simulink model "CubeSat_ADCS"  (R2026a)
settings: Solver=ode4  StopTime=tfinal  FixedStep=1
values from neighbouring files (symbols this model uses):
  A = 0.02    [magnetorquer_params.m]
  Amax = lsort(2)*lsort(3)    [inertia.m]
  AngBias = [1e-4; -2e-4; 1e-4]    [sensor_params.m]
  AngNoise = 1e-4    (= 0.0001)    [sensor_params.m]
  CD = 1.0    (= 1)    [inertia.m]
  desatSpeed = rpm_desat*2*pi/60    (= 104.71975512)    [reaction_wheel_params.m]
  G = 6.67e-11    [planet_params.m]
  Ir1B = T1*IrR*T1'    [reaction_wheel_params.m]
  Ir1Bcg = Ir1B + m_rws*(sr1')*sr1    [reaction_wheel_params.m]
  Ir2B = T2*IrR*T2'    [reaction_wheel_params.m]
  Ir2Bcg = Ir2B + m_rws*(sr2')*sr2    [reaction_wheel_params.m]
  Ir3B = T3*IrR*T3'    [reaction_wheel_params.m]
  Ir3Bcg = Ir3B + m_rws*(sr3')*sr3    [reaction_wheel_params.m]
  Is = (ms/12)*[(ly^2+lz^2) 0 0 ;0 (lx^2+lz^2) 0;0 0 (lx^2+ly^2)]    [inertia.m]
  Jinv = J'/(J*J')    [reaction_wheel_params.m]
  k = 0.001    [Control.m]    (also in Init_Params.m = 67200; main_final.m = (1/6)*(k1+2*k2+2*k3+k4))
  lmax = l(3)    [inertia.m]
  m = ms + 3*m_rws    [inertia.m]
  M = 5.972e24    (= 5.972e+24)    [planet_params.m]
  MagBias = [1e-7; -2e-7; 1.5e-7]    [sensor_params.m]
  MagNoise = 1e-6    (= 1e-06)    [sensor_params.m]
  maxAlpha = maxTorque/IrR(1,1)    [reaction_wheel_params.m]
  maxSpeed = max_rpm*2*pi/60    (= 733.038285838)    [reaction_wheel_params.m]
  n = 84    [magnetorquer_params.m]
  n1 = [1;0;0]    [reaction_wheel_params.m]
  n2 = [0;1;0]    [reaction_wheel_params.m]
  n3 = [0;0;1]    [reaction_wheel_params.m]
  pqr0 = [0.08; -0.02; 0.03]    [Init_Params.m]    (also in main_final.m = [p0; q0; r0])
  q0 = q0123(1)    [Body2ECI_quat.m]    (also in EulerAngles2Quaternions.m = cos(phi/2)*cos(theta/2)*cos(psi/2) + sin(phi/2)*sin(theta/2); Init_Params.m = EulerAngles2Quaternions(ptp0); Quaternions2EulerAngles.m = q0123(:,1); main_final.m = -0.02)
  r0_eci = [x0; y0; z0]    [Init_Params.m]
  s = 0.3    [Init_Params.m]    (also in Navigation.m)
  v0_eci = [0; vcircular*cos(inclination); vcircular*sin(inclination)]    [Init_Params.m]
undefined symbols (not defined in the file or in its folder): IAU
libraries: matrix_library x4, aerolibtransform2 x3, vrlib x3, simulink x3, aerolibutil x1, simulink_extras x1
settings Model: Creator=marca  LastModifiedBy=marca
settings DebuggingCC: SignalInfNanChecking=warning  UnderSpecifiedDimensionMsg=warning

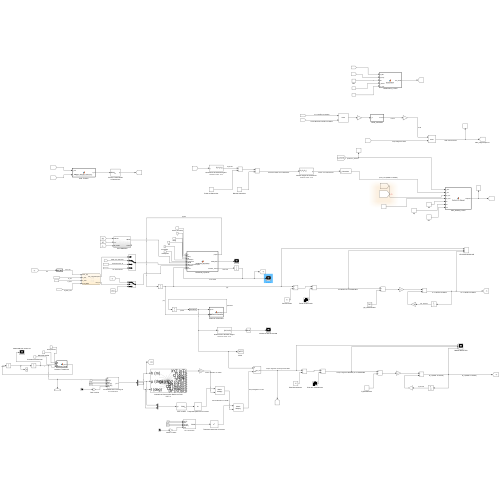
[thumbnail: Simulink's stored preview of the top-level diagram]
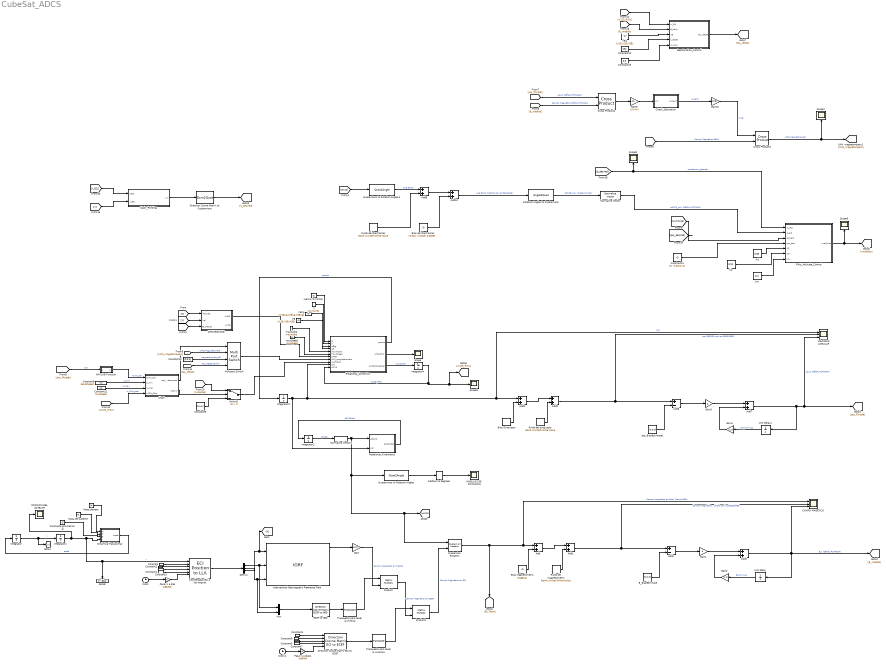
== system CubeSat_ADCS ==
  Add{,1..3,5,7,9..10} (8 alike) : Sum
  Add4 : Sum  Inputs=+-
  Add6 : Sum  Inputs=+-
  B_BiasEstimate : Constant  Value=[0;0;0]
  Bias Giroscopio : Constant  Value=AngBias
  Bias Magnetómetro : Constant  Value=MagBias
  Bias del Startracker : Constant  Value=[0.001; -0.0015; 0.0008]
  CAMPO MAGÉTICO : Scope  NumInputPorts=3
      settings: ActiveDisplayYMinimum=-5.4427960375962918E-5  ActiveDisplayYMaximum=3.9521146554244587E-5  DataLoggingVariableName=ScopeData4
  Chart : Stateflow chart  TreatAsAtomicUnit=on
  Check_Saturation : MATLAB Function  TreatAsAtomicUnit=on
  Clock : Clock
  Clock1 : Clock
  Constant : Constant  Value=0  SampleTime=-1
  Constant{1,3,5,7} (4 alike) : Constant  Value=[0,0]
  Constant10 : Constant  Value=[0;0;0]
  Constant11 : Constant  Value=maxSpeed
  Constant12 : Constant  Value=1e4
  Constant13 : Constant  Value=0.5
  Constant14 : Constant  Value=[0; -0.0011; 0]
  Constant2 : Constant  Value=0
  Constant4 : Constant  Value=0
  Constant6 : Constant  Value=0
  Constant8 : Constant  Value=desatSpeed
  Constant9 : Constant  Value=[0;0;0]
  Constante gravitacional : Constant  Value=G
  Coordenadas ECI a lat-long-alt : aerolibtransform2/ECI Position to LLA  red=IAU-2000/2006  year=2026  month=August  day=1  hour=0  min=0  sec=0  deltaT=Day  errorflag=Error  extraparamflag=on  eunits=Metric (MKS)  earthmodel=WGS84  flat=1/298.257223563  eqradius=6378137
      settings: AttributesFormatString=%<red>
  Cross Product2 : matrix_library/Cross Product
  Cross Product3 : matrix_library/Cross Product
  DISTURBANCE : Subsystem
  Demux : Demux  Outputs=3
  Desaturation_Control : MATLAB Function  TreatAsAtomicUnit=on
  Dinámica Traslacional : MATLAB Function  TreatAsAtomicUnit=on
  Direction Cosine Matrix ECI to ECEF : aerolibtransform2/Direction Cosine Matrix ECI to ECEF  red=IAU-2000/2006  year=2026  month=August  day=1  hour=0  min=0  sec=0  deltaT=Day  errorflag=Error  extraparamflag=on
      settings: AttributesFormatString=%<red>
  Direction Cosine Matrix to Quaternions : Dcm2Quat
  ECEF to NED : aerolibtransform2/Direction Cosine Matrix ECEF to NED
  Gain : Gain  Gain=1e-9
  Gain1 : Gain  Gain=s
  Gain10 : Gain  Gain=n*A
  Gain2 : Gain  Gain=(1-s)
  Gain3 : Gain  Gain=s
  Gain4 : Gain  Gain=(1-s)
  Gain9 : Gain  Gain=k/(n*A)
  Inercia (sin RWs) : Constant  Value=Is
  Integrator : Integrator  InitialCondition=v0_eci
  Integrator1 : Integrator  InitialCondition=r0_eci
  Integrator2 : Integrator  InitialCondition=q0
  Integrator3 : Integrator  InitialCondition=pqr0
  Integrator4 : Integrator  InitialCondition=[0;0;0]
  International Geomagnetic Reference Field : IGRF  time_in=off  month=August  day=1  year=2026
      settings: AttributesFormatString=%<generation>
  IrB : Constant  Value=[Ir1B,Ir2B,Ir3B]
  IrB1 : Constant  Value=[Ir1B,Ir2B,Ir3B]
  IrBcg : Constant  Value=[Ir1Bcg,Ir2Bcg,Ir3Bcg]
  Jinv : Constant  Value=Jinv
  Kd : Constant  Value=0.05
  Kp : Constant  Value=0.01
  MATLAB Function : MATLAB Function  TreatAsAtomicUnit=on
  Masa del satélite : Constant  Value=m
  Masa planeta : Constant  Value=M
  Multiport Switch : MultiPortSwitch  SaturateOnIntegerOverflow=off  InputSameDT=off
  Mux : Mux  Inputs=2
  Nadir_Pointing : MATLAB Function  TreatAsAtomicUnit=on
  Normalize Vector : vrlib/Utilities/Normalize Vector  maxzero=0
  Normalize Vector1 : vrlib/Utilities/Normalize Vector  maxzero=0
  POSICIÓN DEL SATÉLITE : Scope
      settings: ActiveDisplayYMinimum=-8.7137499994663056E+6  ActiveDisplayYMaximum=8.7137499999407E+6
  Pasar s a dias : Gain  Gain=1/86400
  Pasar s a dias1 : Gain  Gain=1/86400
  Product : Product  Multiplication=Matrix(*)
  Product1 : Product  Multiplication=Matrix(*)
  Quaternion Rotation : aerolibutil/Quaternion Rotation
  Quaternions to Rotation Angles : Quat2Angle
      settings: AttributesFormatString=Rotation Order: %<rotationOrder>
  Quaternions to Rotation Angles1 : Quat2Angle
      settings: AttributesFormatString=Rotation Order: %<rotationOrder>
  RWs_Attitude_Control : MATLAB Function  TreatAsAtomicUnit=on
  Radians to Degrees : simulink_extras/Transformations/Radians to Degrees
  Rotation Angles to Quaternions : Angle2Quat
      settings: AttributesFormatString=Rotation Order: %<rotationOrder>
  Rotational_Dynamics : MATLAB Function  TreatAsAtomicUnit=on
  Rotational_Kinematics : MATLAB Function  TreatAsAtomicUnit=on
  Ruido del Startracker : simulink/Sources/Band-Limited White Noise  Cov=[9.4e-9; 9.4e-9; 2.3e-7]  Ts=1  seed=[23341]
  Ruido del giroscopio : simulink/Sources/Band-Limited White Noise  Cov=((AngNoise)^2) * [1; 1; 1]  Ts=1  seed=[23341]
  Ruido del magnetómetro : simulink/Sources/Band-Limited White Noise  Cov=(MagNoise^2) * [1; 1; 1]  Ts=1  seed=[23341]
  Scope{,1..3,5} (5 alike) : Scope
      Scope settings: ActiveDisplayYMinimum=-0.0029922508301770847  ActiveDisplayYMaximum=0.0037761427901097859
      Scope1 settings: ActiveDisplayYMinimum=-1.896452021703556E-8  ActiveDisplayYMaximum=1.737154328387897E-6  DataLoggingVariableName=ScopeData5
      Scope2 settings: ActiveDisplayYMinimum=-0.49886917310286244  ActiveDisplayYMaximum=-0.0070450072202054848  DataLoggingVariableName=ScopeData6
      Scope3 settings: ActiveDisplayYMinimum=-138.56846791071905  ActiveDisplayYMaximum=115.27734503606811  DataLoggingVariableName=ScopeData7
      Scope5 settings: ActiveDisplayYMinimum=-24.785061505875653  ActiveDisplayYMaximum=36.707156844753371  DataLoggingVariableName=ScopeData9
  Switch1 : Switch  Criteria=u2 > Threshold  SaturateOnIntegerOverflow=off  InputSameDT=off
  Traspuesta para tener la inversa : matrix_library/Transpose
  Traspuesta para tener la inversa1 : matrix_library/Transpose
  Unit Delay : UnitDelay  InitialCondition=[0;0;0]  SampleTime=-1
  Unit Delay1 : UnitDelay  InitialCondition=[0;0;0]  SampleTime=-1
  VELCIDAD ANGULAR : Scope  NumInputPorts=3
      settings: ActiveDisplayYMinimum=-0.3287242244754594  ActiveDisplayYMaximum=0.46714614565610874  DataLoggingVariableName=ScopeData3
  maxAlpha : Constant  Value=maxAlpha
  maxSpeed : Constant  Value=maxSpeed
  n : Constant  Value=[n1,n2,n3]
  pqr_BiasEstimate1 : Constant  Value=[0;0;0]
  ÁNGULOS DE ROTACIÓN : Scope
      settings: ActiveDisplayYMinimum=-82.561568673125265  ActiveDisplayYMaximum=52.799854649442857  DataLoggingVariableName=ScopeData2
  wires:
  Integrator/1 -> [v], Integrator1/1  "v"
  Dinámica Traslacional/1(accel) -> Integrator/1  "accel"
  Integrator1/1 -> POSICIÓN DEL SATÉLITE/1, Coordenadas ECI a lat-long-alt/1, [r_ECI], Dinámica Traslacional/4(r)  "r"
  Masa planeta/1 -> Dinámica Traslacional/1(M)
  Masa del satélite/1 -> Dinámica Traslacional/2(m)
  Constante gravitacional/1 -> Dinámica Traslacional/3(G)
  Integrator2/1 -> Normalize Vector1/1  "q0123"
  Inercia (sin RWs)/1 -> Rotational_Dynamics/1(Is)
  Rotational_Dynamics/1(pqrdot) -> Integrator3/1  "pqrdot"
  Integrator3/1 -> Rotational_Kinematics/2(pqr), VELCIDAD ANGULAR/1, Add2/1, Rotational_Dynamics/10(pqr)  "pqr"
  Rotational_Kinematics/1(q0123dot) -> Integrator2/1  "q0123dot"
  Quaternions to Rotation Angles/1 -> Radians to Degrees/1
  Coordenadas ECI a lat-long-alt/1 -> Demux/1
  Demux/1 -> Mux/1, International Geomagnetic Reference Field/2
  Demux/2 -> Mux/2, International Geomagnetic Reference Field/3
  Demux/3 -> [h], International Geomagnetic Reference Field/1
  Constant/1 -> Coordenadas ECI a lat-long-alt/2
  Constant2/1 -> Coordenadas ECI a lat-long-alt/3
  Constant3/1 -> Coordenadas ECI a lat-long-alt/4
  Constant1/1 -> Coordenadas ECI a lat-long-alt/5
  Clock/1 -> Pasar s a dias/1
  Pasar s a dias/1 -> Coordenadas ECI a lat-long-alt/6
  International Geomagnetic Reference Field/1 -> Gain/1
  Gain/1 -> Product/2  "Campo magnético en Teslas"
  Mux/1 -> ECEF to NED/1
  ECEF to NED/1 -> Traspuesta para tener la inversa/1
  Traspuesta para tener la inversa/1 -> Product/1
  Pasar s a dias1/1 -> Direction Cosine Matrix ECI to ECEF/5
  Constant7/1 -> Direction Cosine Matrix ECI to ECEF/3
  Constant4/1 -> Direction Cosine Matrix ECI to ECEF/1
  Constant6/1 -> Direction Cosine Matrix ECI to ECEF/2
  Constant5/1 -> Direction Cosine Matrix ECI to ECEF/4
  Clock1/1 -> Pasar s a dias1/1
  Direction Cosine Matrix ECI to ECEF/1 -> Traspuesta para tener la inversa1/1
  Product/1 -> Product1/2  "Campo Magnético en ECEF"
  Traspuesta para tener la inversa1/1 -> Product1/1
  Product1/1 -> Quaternion Rotation/2  "Campo Magnético en ECI"
  Quaternion Rotation/1 -> CAMPO MAGÉTICO/1, Add/1, [BI_Tesla]  "Campo magnético en Body Frame REAL"
  Bias Magnetómetro/1 -> Add/2
  Add/1 -> Add1/1
  Ruido del magnetómetro/1 -> Add1/2
  Add1/1 -> Add4/1, CAMPO MAGÉTICO/2  "Campo magnético MEDIDO por los SENSORES"
  Add2/1 -> Add3/1
  Ruido del giroscopio/1 -> Add3/2
  Add3/1 -> Add6/1, VELCIDAD ANGULAR/2  "pqr MEDIDA por los SENSORES"
  Bias Giroscopio/1 -> Add2/2
  B_BiasEstimate/1 -> Add4/2
  Add4/1 -> Gain1/1
  Unit Delay/1 -> Gain2/1  "B_kminus1"
  Gain2/1 -> Add5/2
  Gain1/1 -> Add5/1
  Add5/1 -> [B_medido], CAMPO MAGÉTICO/3, Unit Delay/1  "B_k (SEÑAL FILTRADA)"
  Gain4/1 -> Add7/2
  Unit Delay1/1 -> Gain4/1  "pqr_kminus1"
  Add7/1 -> VELCIDAD ANGULAR/3, [pqr_filtrada], Unit Delay1/1  "pqr_k (SEÑAL FILTRADA)"
  pqr_BiasEstimate1/1 -> Add6/2
  Add6/1 -> Gain3/1
  Gain3/1 -> Add7/1
  maxAlpha/1 -> Rotational_Dynamics/5(maxAlpha)
  n/1 -> Rotational_Dynamics/2(n)
  IrB/1 -> Rotational_Dynamics/4(IrB)
  IrBcg/1 -> Rotational_Dynamics/3(IrBcg)
  Rotational_Dynamics/3(w123dot_actual) -> Integrator4/1  "w123_dot"
  Integrator4/1 -> [w123_RWs], Scope3/1, Rotational_Dynamics/11(w123)  "w123_RWs"
  [h] -> DISTURBANCE/1(Altitude)
  [v] -> DISTURBANCE/2(vel)
  [BI_Tesla] -> DISTURBANCE/3(BI_Teslas)
  [q0123] -> Quaternions to Rotation Angles1/1
  Ruido del Startracker/1 -> Add9/2
  Quaternions to Rotation Angles1/1 -> Add9/1  "Ang Euler"
  Add9/1 -> Add10/1
  Bias del Startracker/1 -> Add10/2
  Add10/1 -> Rotation Angles to Quaternions/1  "Ang Euler medido por el Startracker"
  Rotation Angles to Quaternions/1 -> Normalize Vector/1  "q0123_nav (cuaterniones)"
  Normalize Vector/1 -> RWs_Attitude_Control/2(q_act)  "q0123_nav (SEÑAL FILTRADA)"
  [pqr_filtrada] -> RWs_Attitude_Control/3(pqr_act)
  Gain10/1 -> Cross Product3/1  "muB"
  Cross Product3/1 -> Scope1/1, [LMN_magnetorquers]  "LMN_magnetorquers"
  Check_Saturation/1(current) -> Gain10/1  "current"
  [pqr_filtrada] -> Cross Product2/1  "pqr_k (SEÑAL FILTRADA)"
  Gain9/1 -> Check_Saturation/1(i_in)
  Cross Product2/1 -> Gain9/1
  [B_medido] -> Cross Product2/2  "Campo Magnético SEÑAL FILTRADA"
  [BI_Tesla] -> Cross Product3/2  "Campo Magnético REAL"
  Rotational_Dynamics/2(LMN_RWs) -> Scope/1
  maxSpeed/1 -> Rotational_Dynamics/6(maxSpeed)
  DISTURBANCE/1(LMND) -> Rotational_Dynamics/7(LMND)
  [q_desired] -> RWs_Attitude_Control/1(q_des), Scope2/1  "quaternion_desired"
  Radians to Degrees/1 -> ÁNGULOS DE ROTACIÓN/1
  [pqr_filtrada] -> MATLAB Function/1(pqr_filtrada)  "pqr"
  MATLAB Function/1(norm_pqr) -> Chart/1(norm_pqr)  "norm_pqr"
  Chart/2(use_rw) -> Switch1/2
  [LMN_magnetorquers] -> Multiport Switch/2  "LMN_mag_detumble"
  [rwalphas] -> Switch1/1
  Constant9/1 -> Switch1/3
  Multiport Switch/1 -> Rotational_Dynamics/8(LMN_magnetorquers)
  Switch1/1 -> Rotational_Dynamics/9(rwalphas)
  [w123_RWs] -> Chart/4(w123_RWs)  "w_RWs_real"
  Constant8/1 -> Chart/2(w_min)  "w_min"
  Constant11/1 -> Chart/3(w_max)  "w_max"
  Chart/1(use_magnetorquers) -> Multiport Switch/1
  Constant10/1 -> Multiport Switch/3  "magnetorquers_off"
  [w123_RWs] -> Desaturation_Control/1(w_RW)
  [B_medido] -> Desaturation_Control/2(B_body)
  IrB1/1 -> Desaturation_Control/3(IrB)
  Constant12/1 -> Desaturation_Control/4(k_desat)
  Constant13/1 -> Desaturation_Control/5(m_max)
  Desaturation_Control/1(tau_desat) -> [tau_desat]
  [tau_desat] -> Multiport Switch/4  "tau_desaturación"
  [r_ECI] -> Nadir_Pointing/1(r_ECI)
  [v] -> Nadir_Pointing/2(v_ECI)
  [pqr_desired] -> ?
  Normalize Vector1/1 -> Rotational_Kinematics/1(q0123), [q0123], Quaternion Rotation/1, Quaternions to Rotation Angles/1
  Constant14/1 -> RWs_Attitude_Control/4(pqr_des)
  Nadir_Pointing/1(xyz) -> Direction Cosine Matrix to Quaternions/1
  Direction Cosine Matrix to Quaternions/1 -> [q_desired]
  Kd/1 -> RWs_Attitude_Control/5(KP)
  Jinv/1 -> RWs_Attitude_Control/7(Jinv)
  Kp/1 -> RWs_Attitude_Control/6(KD)
  RWs_Attitude_Control/1(rwalphas) -> Scope5/1, [rwalphas]

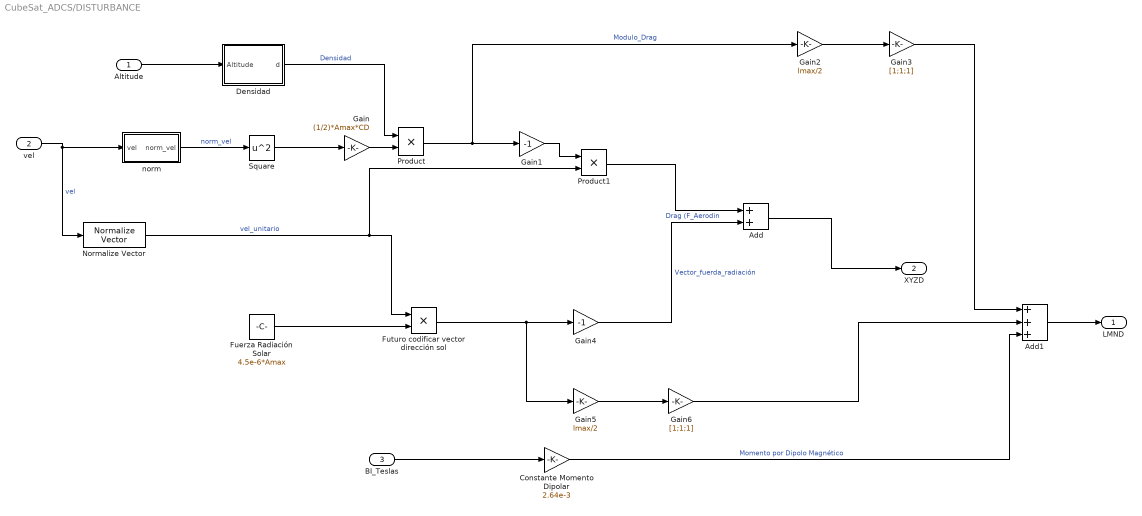
== system CubeSat_ADCS/DISTURBANCE ==
  Altitude : Inport
  vel : Inport  Port=2
  BI_Teslas : Inport  Port=3
  Add : Sum
  Add1 : Sum  Inputs=+++
  Constante Momento Dipolar : Gain  Gain=2.64e-3
  Densidad : MATLAB Function  TreatAsAtomicUnit=on
  Fuerza Radiación Solar : Constant  Value=4.5e-6*Amax
  Futuro codificar vector dirección sol : Product
  Gain : Gain  Gain=(1/2)*Amax*CD
  Gain1 : Gain  Gain=-1
  Gain2 : Gain  Gain=lmax/2
  Gain3 : Gain  Gain=[1;1;1]
  Gain4 : Gain  Gain=-1
  Gain5 : Gain  Gain=lmax/2
  Gain6 : Gain  Gain=[1;1;1]
  Normalize Vector : vrlib/Utilities/Normalize Vector  maxzero=0
  Product : Product
  Product1 : Product
  Square : Math  Operator=square
  norm : MATLAB Function  TreatAsAtomicUnit=on
  LMND : Outport
  XYZD : Outport  Port=2
  wires:
  Altitude/1 -> Densidad/1(Altitude)
  vel/1 -> norm/1(vel), Normalize Vector/1  "vel"
  Normalize Vector/1 -> Futuro codificar vector dirección sol/1, Product1/2  "vel_unitario"
  Gain/1 -> Product/2
  norm/1(norm_vel) -> Square/1  "norm_vel"
  Square/1 -> Gain/1
  Product/1 -> Gain2/1, Gain1/1  "Modulo_Drag"
  Product1/1 -> Add/1  "Drag (F_Aerodin"
  Gain1/1 -> Product1/1
  Add/1 -> XYZD/1
  Gain2/1 -> Gain3/1
  Gain3/1 -> Add1/1
  Add1/1 -> LMND/1
  Fuerza Radiación Solar/1 -> Futuro codificar vector dirección sol/2
  Futuro codificar vector dirección sol/1 -> Gain5/1, Gain4/1
  Gain4/1 -> Add/2  "Vector_fuerda_radiación"
  Gain5/1 -> Gain6/1
  Gain6/1 -> Add1/2
  BI_Teslas/1 -> Constante Momento Dipolar/1
  Constante Momento Dipolar/1 -> Add1/3  "Momento por Dipolo Magnético"
  Densidad/1(d) -> Product/1  "Densidad"

== matlab function CubeSat_ADCS/Nadir_Pointing ==
  data: r_ECI input; xyz output; v_ECI input
function xyz  = Nadir_Attitude_Reference(r_ECI,v_ECI)

%%% NADIR PONTING %%%
% Se tomará el eje +Z como Nadir, el eje Y perpendicular al plano orbital 
% y el eje Z perpendicular a los dos ejes anteriores. 

z = -r_ECI/norm(r_ECI);

y = cross(z, v_ECI);
y = y / norm(y);

x = cross(z,y);

xyz = [x'; y'; z'];

== matlab function CubeSat_ADCS/RWs_Attitude_Control ==
  data: q_des input; rwalphas output; q_act input; pqr_act input; pqr_des input; KP input; KD input; Jinv input
function rwalphas = Control_PD_Robust(q_des, q_act, pqr_act, pqr_des, KP, KD, Jinv)
% 1. Normalización
q_des = q_des / norm(q_des);
q_act = q_act / norm(q_act);

% Asumiendo formato Scalar-First [q0; q1; q2; q3]
q0_d = q_des(1); qv_d = q_des(2:4);
q0_a = q_act(1); qv_a = q_act(2:4);

% 2. Cuaternión Error (q_error = q_des^-1 * q_act)
q0_err = q0_d * q0_a + dot(qv_d, qv_a);
qv_err = q0_d * qv_a - q0_a * qv_d - cross(qv_d, qv_a);

% 3. Corrección Anti-Discontinuidad (Shortest Path)
if q0_err < 0
    qv_err = -qv_err;
end
   
% 4. Error de velocidad angular
pqr_err = pqr_act - pqr_des;

% 5. Par de control y aceleración de ruedas
tau_cmd = - KP * qv_err - KD * pqr_err;
rwalphas = - Jinv * tau_cmd;

== matlab function CubeSat_ADCS/Rotational_Kinematics ==
  data: q0123 input; q0123dot output; pqr input
function q0123dot = Rotational_kinematics(q0123, pqr)
p = pqr(1); q= pqr(2); r = pqr(3);
PQRMAT = [0 -p -q -r;p 0 r -q; q -r 0 p; r q -p 0];
q0123dot = (1/2)*PQRMAT*q0123;

== matlab function CubeSat_ADCS/Dinámica Traslacional ==
  data: M input; m input; G input; r input; accel output
function accel = Translational_Dynamics(M,m,G,r)
r = r(:);
rho = norm(r);
r_unit = r/rho; 
Fgrav = -(G*M*m/rho^2)*r_unit; 

accel = Fgrav/m;

== matlab function CubeSat_ADCS/Rotational_Dynamics ==
  data: pqrdot output size=[3 1]; LMN_RWs output size=[3 1]; w123dot_actual output size=[3 1]; Is input size=[3 3]; n input size=[3 3]; IrBcg input size=[3 9]; IrB input size=[3 9]; maxAlpha input size=[1 1]; maxSpeed input; LMND input size=[3 1]; LMN_magnetorquers input size=[3 1]; rwalphas input size=[3 1]; pqr input size=[3 1]; w123 input size=[3 1]
function [pqrdot, LMN_RWs, w123dot_actual] = Rotational_Dynamics(Is, n, IrBcg, IrB, maxAlpha,maxSpeed,LMND,LMN_magnetorquers,rwalphas,pqr,w123)

% Pre-asignación para asegurar dimensiones fijas 3x1 en Simulink
pqrdot = zeros(3,1);
LMN_RWs = zeros(3,1);
w123dot_actual = zeros(3,1);

% Vectores de dirección (3x1)
n1 = n(:,1);
n2 = n(:,2);
n3 = n(:,3);

% Extraer las MATRICES 3x3 completas desde las entradas 3x9
Ir1B = IrB(:, 1:3);
Ir2B = IrB(:, 4:6);
Ir3B = IrB(:, 7:9);

Ir1Bcg = IrBcg(:, 1:3);
Ir2Bcg = IrBcg(:, 4:6);
Ir3Bcg = IrBcg(:, 7:9);

% Inercia total sumada (3x3)
I = Is + Ir1Bcg + Ir2Bcg + Ir3Bcg;
invI = inv(I);

% Limitación de aceleración por hardware
% Limitación de aceleración y velocidad por hardware (CORREGIDO)
for idx = 1:3
    % Si superó la velocidad máxima Y la aceleración solicitada tiene el MISMO signo (busca acelerar más):
    if abs(w123(idx)) >= maxSpeed && (sign(rwalphas(idx)) == sign(w123(idx)) || rwalphas(idx) == 0)
        w123dot_actual(idx) = 0; % Impide seguir acelerando
    elseif abs(rwalphas(idx)) > maxAlpha
        w123dot_actual(idx) = sign(rwalphas(idx)) * maxAlpha;
    else
        w123dot_actual(idx) = rwalphas(idx); % Permite frenar/desacelerar libremente
    end
end

% Par de las ruedas (Identico a tu script: Matriz 3x3 * Escalar * Vector 3x1 = Vector 3x1)
LMN_RWs = Ir1B * (w123dot_actual(1) * n1) + ...
          Ir2B * (w123dot_actual(2) * n2) + ...
          Ir3B * (w123dot_actual(3) * n3);

% Par Neto sobre la estructura (3x1)
LMN = LMN_magnetorquers - LMN_RWs + LMND;

% Momento angular acumulado (Identico a tu script)
w1 = w123(1);
w2 = w123(2);
w3 = w123(3);
H = Is * pqr + Ir1Bcg * (w1 * n1) + Ir2Bcg * (w2 * n2) + Ir3Bcg * (w3 * n3);

% Ecuación de Euler (3x1)
pqrdot = invI * (LMN - cross(pqr, H));

== matlab function CubeSat_ADCS/DISTURBANCE/Densidad ==
  data: Altitude input; d output
function d = fcn(Altitude)
ds = 1.225; %%kg/m^3
sigma = 0.1354; %%scale height;
d = ds * exp(-sigma*Altitude/1000);

== matlab function CubeSat_ADCS/DISTURBANCE/norm ==
  data: vel input; norm_vel output
function norm_vel = fcn(vel)

norm_vel = norm(vel);

== matlab function CubeSat_ADCS/Check_Saturation ==
  data: i_in input; current output
function current = current_saturation(i_in)
maxCurrent = 0.04; % 40 mA
current = i_in;
if sum(abs(i_in)) > maxCurrent
    current = (i_in/ norm(i_in)) * maxCurrent;
end

== stateflow chart CubeSat_ADCS/Chart ==
  state DETUMBLE
    entry:
    use_magnetorquers = 1;
    use_rw = 0;
  state ATTITUDE_CONTROL
    entry:
    use_magnetorquers = 2;
    use_rw = 1;
  state DESATURATION
    entry:
    use_magnetorquers = 3
    use_rw = 1
  (default) -> DETUMBLE
  DETUMBLE -> ATTITUDE_CONTROL : [norm_pqr<0.01]
  ATTITUDE_CONTROL -> DESATURATION : [max(abs(w123_RWs)) > 0.9*w_max && after(500, sec)]
  DESATURATION -> ATTITUDE_CONTROL : [max(abs(w123_RWs)) < w_min && after(10, sec)]
  data: use_magnetorquers output; use_rw output; norm_pqr input; w_min input; w_max input; w123_RWs input

== matlab function CubeSat_ADCS/MATLAB Function ==
  data: pqr_filtrada input; norm_pqr output
function norm_pqr = norm(pqr_filtrada)

norm_pqr = norm(pqr_filtrada);

== matlab function CubeSat_ADCS/Desaturation_Control ==
  data: w_RW input; tau_desat output; B_body input; IrB input; k_desat input; m_max input
function tau_desat = desaturation(w_RW, B_body, IrB, k_desat, m_max)
% w_RW: Velocidad angular de las ruedas (3x1) [rad/s]
% B_body: Campo magnético medido en Body Frame (3x1) [T]
% IrB: Inercia de las ruedas (3x1 o escalar)
% k_desat: Ganancia de desaturación
% m_max: Momento dipolar máximo del magnetopar [A*m^2]
% 1. Extraer matrices de inercia 3x3 individuales
Ir1B = IrB(1:3, 1:3);
Ir2B = IrB(1:3, 4:6);
Ir3B = IrB(1:3, 7:9);

% 2. Momento angular total sumando el aporte de las 3 ruedas
H_RW = Ir1B*[w_RW(1);0;0] + Ir2B*[0;w_RW(2);0] + Ir3B*[0;0;w_RW(3)];

% 3. Momento dipolar requerido para frenar las ruedas
m_req = -k_desat * cross(H_RW, B_body);

% 4. Saturación por hardware del magnetopar
m_act = min(max(m_req, -m_max), m_max);

% 5. Torque magnético resultante sobre la estructura del satélite
tau_desat = -cross(m_act, B_body);
